simulink model "targetVehicle"  (R2015b)
settings: Solver=FixedStepAuto  SolverMode=SingleTasking  StartTime=0.0  StopTime=10.0  FixedStep=0.005  RelTol=1e-3
undefined symbols (not defined in the file): targetPosition, targetVelocity
settings Model: Creator=Josef  LastModifiedBy=Josef
settings OptimizationCC: BlockReduction=off
settings DebuggingCC: SaveWithParameterizedLinksMsg=none
settings HardwareCC: ProdBitPerPointer=32  ProdWordSize=32  ProdHWDeviceType=Intel->x86-32 (Windows32)
settings ModelReferenceCC: ModelReferenceMinAlgLoopOccurrences=on

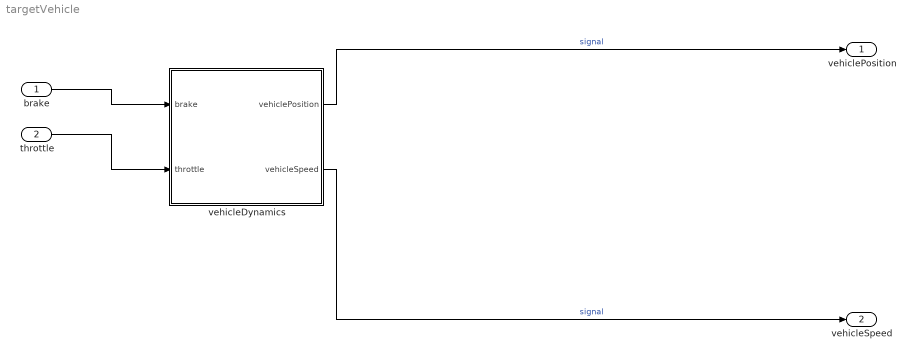
== system targetVehicle ==
  brake : Inport
  throttle : Inport  Port=2
  vehicleDynamics : Subsystem  Variant=on  OverrideUsingVariant=truck
  vehiclePosition : Outport
      settings: AttributesFormatString=signal
  vehicleSpeed : Outport  Port=2
      settings: AttributesFormatString=signal
  wires:
  vehicleDynamics/1(vehiclePosition) -> vehiclePosition/1  "signal"
  vehicleDynamics/2(vehicleSpeed) -> vehicleSpeed/1  "signal"
  throttle/1 -> vehicleDynamics/2(throttle)
  brake/1 -> vehicleDynamics/1(brake)

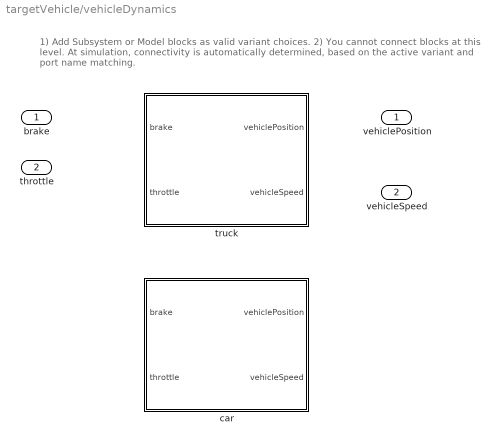
== system targetVehicle/vehicleDynamics ==
  note: 1) Add Subsystem or Model blocks as valid variant choices.
      | 2) You cannot connect blocks at this level. At simulation, connectivity is automatically
      | determined, based on the active variant and port name matching.
  brake : Inport
  throttle : Inport  Port=2
  car : Subsystem  VariantControl=car
  truck : Subsystem  VariantControl=truck
  vehiclePosition : Outport
  vehicleSpeed : Outport  Port=2

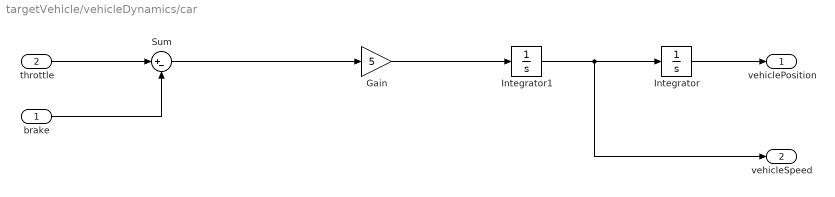
== system targetVehicle/vehicleDynamics/car ==
  brake : Inport
  throttle : Inport  Port=2
  Gain : Gain  Gain=5
  Integrator : Integrator  InitialCondition=targetPosition
  Integrator1 : Integrator  InitialCondition=targetVelocity
  Sum : Sum  Inputs=|+-
  vehiclePosition : Outport
      settings: AttributesFormatString=signal
  vehicleSpeed : Outport  Port=2
      settings: AttributesFormatString=signal
  wires:
  brake/1 -> Sum/2
  throttle/1 -> Sum/1
  Sum/1 -> Gain/1
  Gain/1 -> Integrator1/1
  Integrator1/1 -> Integrator/1, vehicleSpeed/1
  Integrator/1 -> vehiclePosition/1

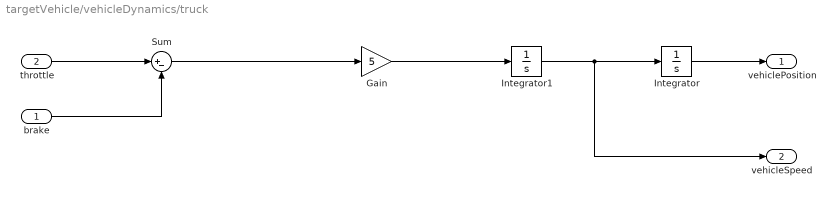
== system targetVehicle/vehicleDynamics/truck ==
  brake : Inport
  throttle : Inport  Port=2
  Gain : Gain  Gain=5
  Integrator : Integrator  InitialCondition=targetPosition
  Integrator1 : Integrator  InitialCondition=targetVelocity
  Sum : Sum  Inputs=|+-
  vehiclePosition : Outport
      settings: AttributesFormatString=signal
  vehicleSpeed : Outport  Port=2
      settings: AttributesFormatString=signal
  wires:
  Integrator/1 -> vehiclePosition/1
  Integrator1/1 -> vehicleSpeed/1, Integrator/1
  Gain/1 -> Integrator1/1
  Sum/1 -> Gain/1
  throttle/1 -> Sum/1
  brake/1 -> Sum/2
